simulink model "ModelTests"  (R2017a)
settings: Solver=FixedStepAuto  StartTime=0.0  StopTime=100  FixedStep=0.01  RelTol=1e-3
libraries: cstblocks x1
settings Model: Creator=roman  LastModifiedBy=roman

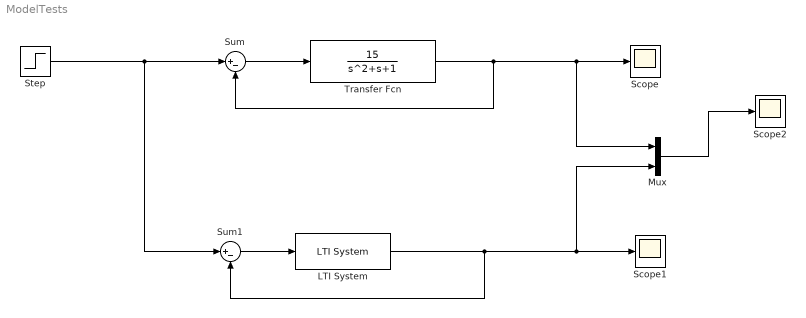
== system ModelTests ==
  LTI System : cstblocks/LTI System  sys=ss1  IC=[]
  Mux : Mux  Inputs=2
  Scope : Scope
  Scope1 : Scope
  Scope2 : Scope
  Step : Step  SampleTime=0
  Sum : Sum  Inputs=|+-
  Sum1 : Sum  Inputs=|+-
  Transfer Fcn : TransferFcn  Numerator=[15]  Denominator=[1 1 1]
  wires:
  Transfer Fcn/1 -> Sum/2, Scope/1, Mux/1
  Step/1 -> Sum1/1, Sum/1
  Sum/1 -> Transfer Fcn/1
  Sum1/1 -> LTI System/1
  Mux/1 -> Scope2/1
  LTI System/1 -> Scope1/1, Mux/2, Sum1/2
